simulink model "salaDeAula"  (R2018b)
settings: Solver=VariableStepAuto  StartTime=0.0  StopTime=100.0  RelTol=1e-3
values from neighbouring files (symbols this model uses):
  alpha = 1*pi/180    (= 0.0174532925199)    [setup.m]
  b = DH/roCp    (= -11.92)    [fsolve1.m]    (also in setup.m = 7)
  c = UA/roCp/V    (= 0.3)    [fsolve1.m]    (also in setup.m = 3)
  g = 9.8    [setup.m]
  m = 1200    [setup.m]
settings Model: Creator=marcelo  LastModifiedBy=marcelo

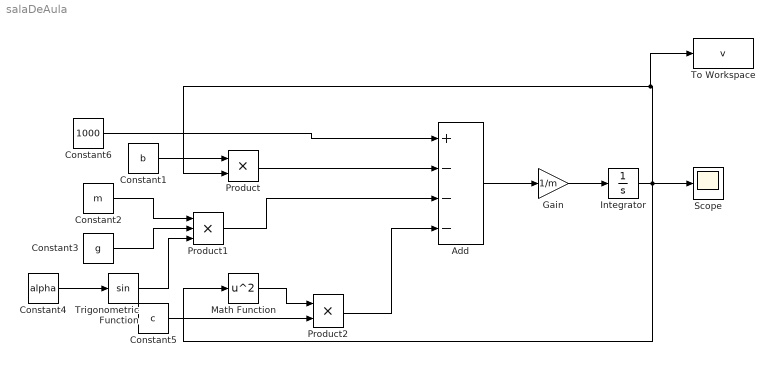
== system salaDeAula ==
  Add : Sum  Inputs=+---
  Constant1 : Constant  Value=b
  Constant2 : Constant  Value=m
  Constant3 : Constant  Value=g
  Constant4 : Constant  Value=alpha
  Constant5 : Constant  Value=c
  Constant6 : Constant  Value=1000
  Gain : Gain  Gain=1/m
  Integrator : Integrator
  Math Function : Math  Operator=square  SaturateOnIntegerOverflow=on
  Product : Product
  Product1 : Product  Inputs=3
  Product2 : Product
  Scope : Scope
  To Workspace : ToWorkspace  VariableName=v  SaveFormat=Timeseries  SampleTime=-1
  Trigonometric Function : Trigonometry
  wires:
  Product/1 -> Add/2
  Constant1/1 -> Product/1
  Product1/1 -> Add/3
  Constant2/1 -> Product1/1
  Constant3/1 -> Product1/2
  Constant5/1 -> Product2/2
  Math Function/1 -> Product2/1
  Product2/1 -> Add/4
  Add/1 -> Gain/1
  Gain/1 -> Integrator/1
  Integrator/1 -> Scope/1, To Workspace/1, Product/2, Math Function/1
  Constant4/1 -> Trigonometric Function/1
  Trigonometric Function/1 -> Product1/3
  Constant6/1 -> Add/1
